simulink model "pll_model"  (R2012b)
settings: Solver=FixedStepDiscrete  StartTime=0.0  StopTime=0.2  RelTol=1e-3
InitFcn:
  | clear_simulation
StartFcn:
  | open_scopes
settings Model: Creator=Tomasz  LastModifiedBy=tomas_000

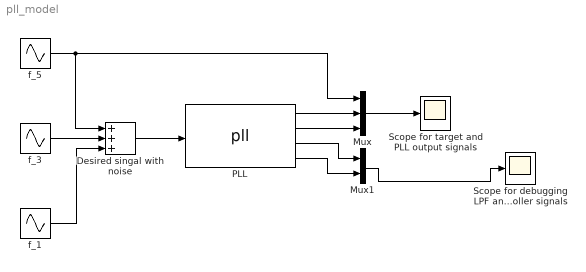
== system pll_model ==
  Desired singal with noise : Sum  Inputs=+++
  Mux : Mux  Inputs=3
  Mux1 : Mux  Inputs=2
  PLL : S-Function  InitFcn=try, set_param(gcb,'FunctionName','pll'), end  FunctionName=pll  SFunctionModules=pll_wrapper low_pass_filter pi_controller saw_tooth_generator  EnableBusSupport=off  mask(S-Function Builder){}
      mask help: Simulink:masks:SFunctionBuilder_MD
      mask init:
      | val = [[.9  0.75 0.75 1 1 .9 .9 1]',[1 1 0.75 0.75 .9 .9 1 .9]'];try , sys = get_param(gcb,'SfunBuilderFcnName');if isempty(sys), sys = get_param(gcb,'FunctionName'); end,catch, sys = get_param(gcb,'FunctionName'); end
      settings: CopyFcn=set_param(gcbh,'LinkStatus','none')  PreSaveFcn=try, set_param(gcb,'FunctionName','pll'), end  OpenFcn=sfunctionwizard(gcbh)
      mask Display: plot(val(:,1),val(:,2)),disp(sys), port_label('input',1,'signal_in'), port_label('output',1,'pll_out'), port_label('output',2,'saw_out'), port_label('output',3,'lpf_out'), port_label('output',4,'pi_ctrl_out')
  Scope for target and PLL output signals : Scope
      settings: ShowLegends=on  YMin=-1  YMax=6.5  MaxDataPoints=1e4
  Scope for debugging LPF and PI controller signals : Scope
      settings: ShowLegends=on  YMin=-0.1  YMax=1.2  MaxDataPoints=1e4
  f_1 : Sin  Frequency=50 * 2 * pi  Phase=5 / 180 * pi  SampleTime=1e-4
  f_3 : Sin  Frequency=150 * 2 * pi  Phase=10 / 180 * pi  SampleTime=1e-4
  f_5 : Sin  Frequency=250 * 2 * pi  Phase=30 / 180 * pi  SampleTime=1e-4
  wires:
  f_5/1 -> Desired singal with noise/1, Mux/1
  f_3/1 -> Desired singal with noise/2
  f_1/1 -> Desired singal with noise/3
  Desired singal with noise/1 -> PLL/1
  PLL/1 -> Mux/2
  Mux/1 -> Scope for target and PLL output signals/1
  Mux1/1 -> Scope for debugging LPF and PI controller signals/1
  PLL/4 -> Mux1/2
  PLL/2 -> Mux/3
  PLL/3 -> Mux1/1
